simulink model "blockdemo"  (Simulink 6.3)
settings: Solver=FixedStepDiscrete  StartTime=0.0  StopTime=10.0  RelTol=1e-3
InitFcn:
  | %% DSPBuilder Start
  | alt_dspbuilder_update_model(bdroot)
  | %% DSPBuilder End
libraries: allblocks_alteradspbuilder2 x5
settings Model: LastModifiedBy=delphick

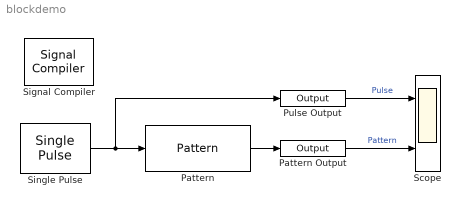
== system blockdemo ==
  Pattern : allblocks_alteradspbuilder2/Pattern  Sequence=10  SpecifyClock=off  use_ena=off  use_sclr=on
  Pattern Output : allblocks_alteradspbuilder2/Output  iofile=C:\workspace_clean\Documentation\DesignExamples\Tutorials\UnitBlocks\GateAndControl\SinglePulse\tb_blockdemo\blockdemo_Pattern+Output.capture  BusType=Single Bit  bwl=8  bwr=0  PORTTYPE=Output
  Pulse Output : allblocks_alteradspbuilder2/Output  iofile=C:\workspace_clean\Documentation\DesignExamples\Tutorials\UnitBlocks\GateAndControl\SinglePulse\tb_blockdemo\blockdemo_Pulse+Output.capture  BusType=Single Bit  bwl=8  bwr=0  PORTTYPE=Output
  Scope : Scope  NumInputPorts=2
      settings: TimeRange=10  YMin=-2~-2  YMax=2~2
  Signal Compiler : allblocks_alteradspbuilder2/Signal Compiler  DeviceFamily=Stratix IV  DeviceName=AUTO  EnableSignalTap=off  SignalTapDepth=128  UseBoardBlock=off  StpUseDefaultClock=on  StpClock=clock
  Single Pulse : allblocks_alteradspbuilder2/Single Pulse  signal_type=Step Down  impulse_width=1  delay=1  SpecifyClock=off  use_ena=off  use_sclr=off
  wires:
  Single Pulse/1 -> Pattern/1, Pulse Output/1
  Pattern/1 -> Pattern Output/1
  Pulse Output/1 -> Scope/1  "Pulse"
  Pattern Output/1 -> Scope/2  "Pattern"
